simulink model "untitled"  (R2014b)
settings: Solver=ode23t  StartTime=0.0  StopTime=10.0  RelTol=1e-3
libraries: powerlib x8, powerlib_meascontrol x6
settings Model: Creator=Khalil  LastModifiedBy=Khalil

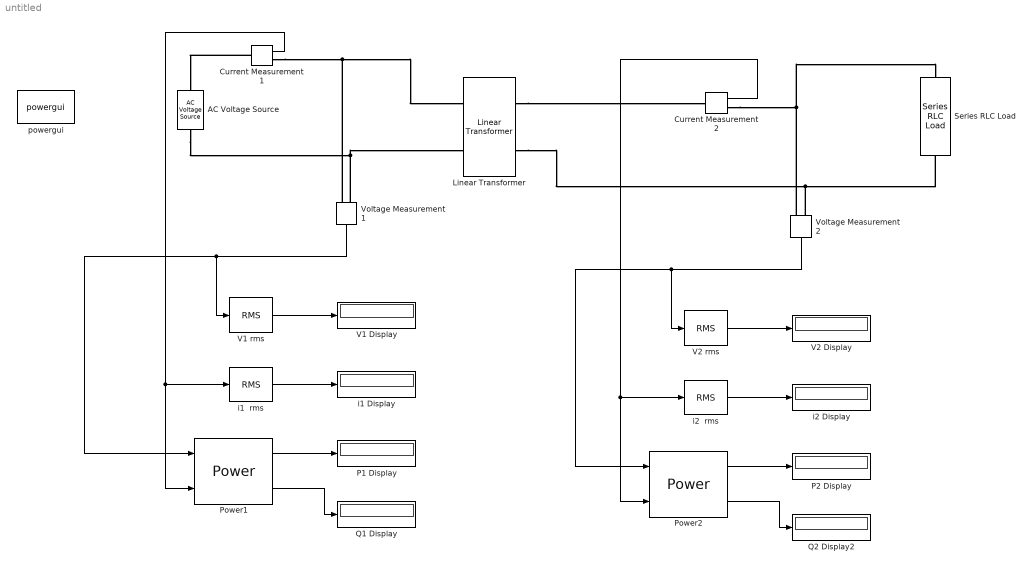
== system untitled ==
  " V1 Display" : Display
  " V2 Display" : Display
  " i1 Display" : Display
  " i2 Display" : Display
  AC Voltage Source : powerlib/Electrical Sources/AC Voltage Source  Amplitude=970*sqrt(2)  Phase=0  Frequency=50  SampleTime=0  Measurements=None
  Current Measurement 1 : powerlib/Measurements/Current Measurement  PhasorSimulation=off  OutputType=Complex  PSBequivalent=0
  Current Measurement 2 : powerlib/Measurements/Current Measurement  PhasorSimulation=off  OutputType=Complex  PSBequivalent=0
  Linear Transformer : powerlib/Elements/Linear Transformer  UNITS=SI  NominalPower=[16750 50]  winding1=[970 1.40432835820896 0.00447238330639795]  winding2=[194 0.0877705223880597 0.000279523956649872]  ThreeWindings=off  winding3=[3.15e+05 0.7938 0.084225]  RmLm=[2808.65671641791 13.4171499191938]  Measurements=None  DataType=on
  P1 Display : Display
      settings: Format=decimal (Stored Integer)
  P2 Display : Display
      settings: Format=decimal (Stored Integer)
  Power1 : powerlib_meascontrol/Measurements/Power  Freq=50  Vinit=[1, 0]  Iinit=[1, 0]  Ts=0
  Power2 : powerlib_meascontrol/Measurements/Power  Freq=50  Vinit=[1, 0]  Iinit=[1, 0]  Ts=0
  Q1 Display : Display
      settings: Format=decimal (Stored Integer)
  Q2 Display2 : Display
      settings: Format=decimal (Stored Integer)
  Series RLC Load : powerlib/Elements/Series RLC Load  LConnTagsString=a  RConnTagsString=__new0  NominalVoltage=194  NominalFrequency=50  ActivePower=0  InductivePower=16750  CapacitivePower=0  Setx0=off  InitialVoltage=0  SetiL0=off  InitialCurrent=0  Measurements=None
  "V1 rms " : powerlib_meascontrol/Measurements/RMS  TrueRMS=on  Freq=50  RMSInit=120  Ts=0
  "V2 rms " : powerlib_meascontrol/Measurements/RMS  TrueRMS=on  Freq=50  RMSInit=120  Ts=0
  Voltage Measurement 1 : powerlib/Measurements/Voltage Measurement  PhasorSimulation=off  OutputType=Complex  PSBequivalent=0
  Voltage Measurement 2 : powerlib/Measurements/Voltage Measurement  PhasorSimulation=off  OutputType=Complex  PSBequivalent=0
  i1  rms : powerlib_meascontrol/Measurements/RMS  TrueRMS=on  Freq=50  RMSInit=120  Ts=0
  i2  rms : powerlib_meascontrol/Measurements/RMS  TrueRMS=on  Freq=50  RMSInit=120  Ts=0
  powergui : powerlib/powergui  Priority=1  SimulationMode=Continuous  SolverType=Tustin/Backward Euler (TBE)  SampleTime=50e-6  frequency=60  SPID=off  DisableSnubberDevices=off  DisableRonSwitches=off  DisableVfSwitches=off  SwTol=0  DisplayEquations=off  Interpol=off  methode=off  Ts=100  frequencyindice=50  Pbase=100e6  ErrMax=1e-4  Iterations=50  UnitsV=kV  UnitsW=MW  FunctionMessages=off  echomessages=off  HookPort=off  EnableUseOfTLC=off  x0status=blocks  RestoreLinks=warning  ResistiveCurrentMeasurement=off  Frange=[0:2:500]  Ylog=off  Xlog=on  ShowGrid=off  save=off  variable=ZData  structure=0  ZoomFFT=off  StartTime=0.0  cycles=1  DisplayStyle=1  fundamental=60  FreqAxis=off  MaxFrequency=1000  frequencyindicesteady=1  RmsSteady=1  display=off
  wires:
  Current Measurement 1/1 -> i1  rms/1, Power1/2
  Voltage Measurement 1/1 -> "V1 rms "/1, Power1/1
  "V1 rms "/1 -> " V1 Display"/1
  i1  rms/1 -> " i1 Display"/1
  Power1/1 -> P1 Display/1
  Power1/2 -> Q1 Display/1
  Current Measurement 2/1 -> i2  rms/1, Power2/2
  Voltage Measurement 2/1 -> "V2 rms "/1, Power2/1
  "V2 rms "/1 -> " V2 Display"/1
  i2  rms/1 -> " i2 Display"/1
  Power2/1 -> P2 Display/1
  Power2/2 -> Q2 Display2/1
  connections:
  Current Measurement 1/LConn1 -- AC Voltage Source/RConn1
  Current Measurement 1/RConn1 -- Voltage Measurement 1/LConn1 -- Linear Transformer/LConn1
  AC Voltage Source/LConn1 -- Linear Transformer/LConn2 -- Voltage Measurement 1/LConn2
  Linear Transformer/RConn2 -- Series RLC Load/RConn1 -- Voltage Measurement 2/LConn2
  Linear Transformer/RConn1 -- Current Measurement 2/LConn1
  Current Measurement 2/RConn1 -- Series RLC Load/LConn1 -- Voltage Measurement 2/LConn1
